simulink model "attitude_interface_sequence"  (R2019b)
settings: Solver=FixedStepAuto  StartTime=0.0  StopTime=inf  FixedStep=FIXED_STEP_SIZE  RelTol=1e-3
model workspace (MAT data in the model file):
  K_ip = 0
  K_pp = 3
values from neighbouring files (symbols this model uses):
  DEG2RAD = pi/180    (= 0.0174532925199)    [attitude_interface_main.m]
  FIXED_STEP_SIZE = 0.01    [attitude_interface_main.m]
  GAZEBO_SYNC_DT = 0.01    [attitude_interface_main.m]
  RAD2DEG = 180/pi    (= 57.2957795131)    [attitude_interface_main.m]
  THRUST_OFFSET = 7.16    [attitude_interface_main.m]
undefined symbols (not defined in the file or in its folder): Header, Pitch, Roll, Thrust, YawRate
libraries: robotlib x5, simulink x3, robotgazebolib x1
settings Model: Creator=ananda  LastModifiedBy=dennis
settings OptimizationCC: EnhancedBackFolding=on  PassReuseOutputArgsAs=Individual arguments  ZeroExternalMemoryAtStartup=off  ZeroInternalMemoryAtStartup=off  MaxStackSize=64  OptimizeBlockOrder=speed  DifferentSizesBufferReuse=on  OptimizationCustomize=off  EfficientTunableParamExpr=on
settings DebuggingCC: ParameterTunabilityLossMsg=error
settings HardwareCC: ProdBitPerPointer=32  ProdBitPerSizeT=32  ProdBitPerPtrDiffT=32  ProdLargestAtomicFloat=None  ProdIntDivRoundTo=Undefined  ProdEndianess=Unspecified  ProdWordSize=32  ProdHWDeviceType=Generic->Unspecified (assume 32-bit Generic)  UseEmbeddedCoderFeatures=off
settings SFSimCC: MATLABDynamicMemAlloc=off
settings RTWCC: SystemTargetFile=ert.tlc  HardwareBoard=Robot Operating System (ROS)  TLCOptions="-aInlineSetEventsForThisBaseRateFcn=TLC_FALSE -aSuppressMultiTaskScheduler=TLC_FALSE  -aRateBasedStepFcn=0"  TemplateMakefile=ert_default_tmf  GenerateReport=on  Toolchain=Catkin  IncludeHyperlinkInReport=on  LaunchReport=on  TargetLang=C++  GenerateTraceInfo=on  GenerateTraceReport=on  GenerateTraceReportSl=on  GenerateTraceReportSf=on  GenerateTraceReportEml=on
settings CodeAppCC: ForceParamTrailComments=on  IgnoreCustomStorageClasses=off  OperatorAnnotations=on  SimulinkDataObjDesc=on  SFDataObjDesc=on  InsertBlockDesc=on
settings ERTTargetCC: SupportNonInlinedSFcns=on

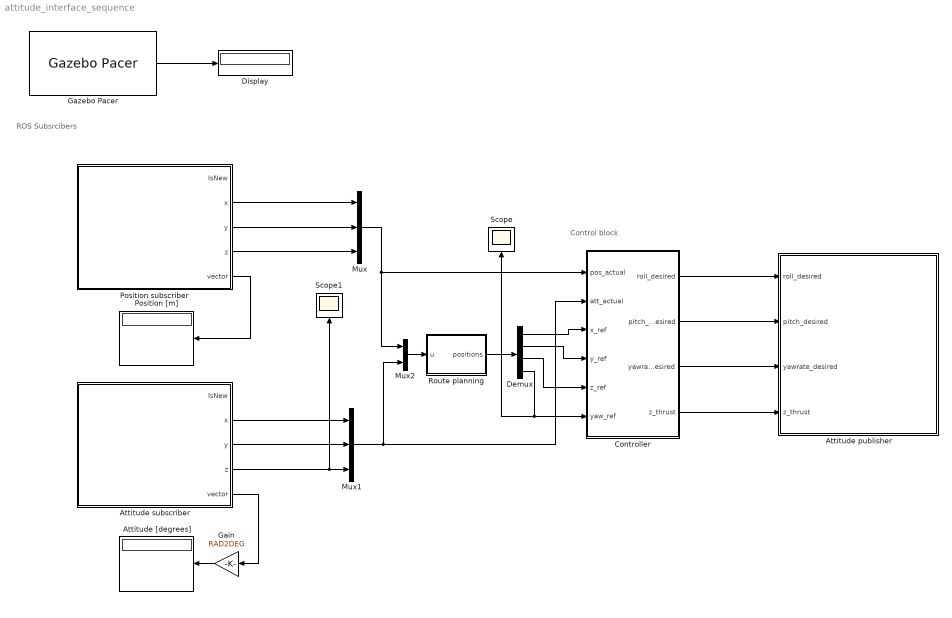
== system attitude_interface_sequence ==
  note: Control block
  note: ROS Subsrcibers
  Attitude [degrees] : Display
  Attitude publisher : Subsystem
  Attitude subscriber : Subsystem
  Controller : Subsystem
  Demux : Demux
  Display : Display
  Gain : Gain  Gain=RAD2DEG
  Gazebo Pacer : robotgazebolib/Gazebo Pacer  ResetBehavior=Reset Gazebo simulation time  SampleTime=GAZEBO_SYNC_DT
      settings: SourceProductName=Robotics System Toolbox  SourceProductBaseCode=RO
  Mux : Mux  Inputs=3
  Mux1 : Mux  Inputs=3
  Mux2 : Mux  Inputs=2
  Position [m] : Display
  Position subscriber : Subsystem
  Route planning : MATLAB Function  TreatAsAtomicUnit=on
      settings: MinAlgLoopOccurrences=on
  Scope : Scope
  Scope1 : Scope
  wires:
  Position subscriber/5(vector) -> Position [m]/1
  Attitude subscriber/5(vector) -> Gain/1
  Gain/1 -> Attitude [degrees]/1
  Gazebo Pacer/1 -> Display/1
  Controller/1(roll_desired) -> Attitude publisher/1(roll_desired)
  Controller/2(pitch_desired) -> Attitude publisher/2(pitch_desired)
  Controller/3(yawrate_desired) -> Attitude publisher/3(yawrate_desired)
  Controller/4(z_thrust) -> Attitude publisher/4(z_thrust)
  Attitude subscriber/2(x) -> Mux1/1
  Attitude subscriber/3(y) -> Mux1/2
  Attitude subscriber/4(z) -> Mux1/3, Scope1/1
  Position subscriber/4(z) -> Mux/3
  Position subscriber/3(y) -> Mux/2
  Position subscriber/2(x) -> Mux/1
  Mux/1 -> Mux2/1, Controller/1(pos_actual)
  Mux1/1 -> Mux2/2, Controller/2(att_actual)
  Mux2/1 -> Route planning/1(u)
  Route planning/1(positions) -> Demux/1
  Demux/1 -> Controller/3(x_ref)
  Demux/2 -> Controller/4(y_ref)
  Demux/3 -> Controller/5(z_ref)
  Demux/4 -> Controller/6(yaw_ref), Scope/1

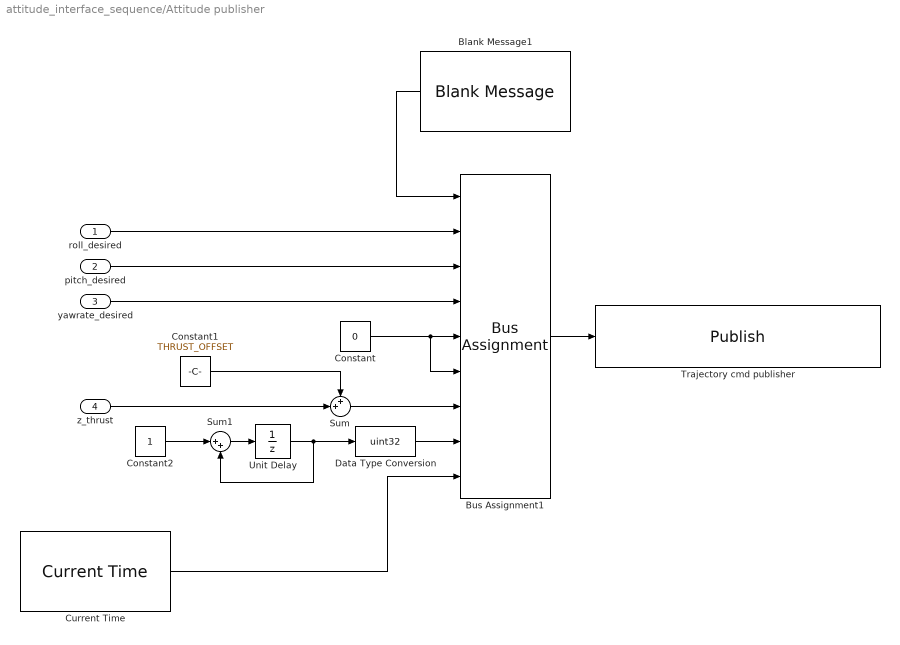
== system attitude_interface_sequence/Attitude publisher ==
  roll_desired : Inport
  pitch_desired : Inport  Port=2
  yawrate_desired : Inport  Port=3
  z_thrust : Inport  Port=4
  Blank Message1 : robotlib/Blank Message  messageClass=Message  entityType=mav_msgs/RollPitchYawrateThrust  messageType=mav_msgs/RollPitchYawrateThrust  SampleTime=FIXED_STEP_SIZE
      settings: SourceProductName=ROS Toolbox
  Bus Assignment1 : BusAssignment  AssignedSignals=Roll,Pitch,YawRate,Thrust.X,Thrust.Y,Thrust.Z,Header.Seq,Header.Stamp
  Constant : Constant  Value=0
  Constant1 : Constant  Value=THRUST_OFFSET
  Constant2 : Constant
  Current Time : robotlib/Current Time  OutputFormat=bus  SampleTime=FIXED_STEP_SIZE  ModelName=attitude_interface_sequence
      settings: SourceProductName=ROS Toolbox  SourceProductBaseCode=RR
  Data Type Conversion : DataTypeConversion  OutDataTypeStr=uint32
  Sum : Sum  Inputs=++|
  Sum1 : Sum  Inputs=|++
  Trajectory cmd publisher : robotlib/Publish  topicSource=Specify your own  topic=/hummingbird/command/roll_pitch_yawrate_thrust  messageType=mav_msgs/RollPitchYawrateThrust  messageQueueLength=1
      settings: SourceProductName=ROS Toolbox
  Unit Delay : UnitDelay  SampleTime=FIXED_STEP_SIZE  HasFrameUpgradeWarning=on
  wires:
  Bus Assignment1/1 -> Trajectory cmd publisher/1
  Blank Message1/1 -> Bus Assignment1/1
  Constant/1 -> Bus Assignment1/6, Bus Assignment1/5
  yawrate_desired/1 -> Bus Assignment1/4
  pitch_desired/1 -> Bus Assignment1/3
  roll_desired/1 -> Bus Assignment1/2
  Sum/1 -> Bus Assignment1/7
  z_thrust/1 -> Sum/2
  Constant1/1 -> Sum/1
  Sum1/1 -> Unit Delay/1
  Unit Delay/1 -> Sum1/2, Data Type Conversion/1
  Constant2/1 -> Sum1/1
  Current Time/1 -> Bus Assignment1/9
  Data Type Conversion/1 -> Bus Assignment1/8

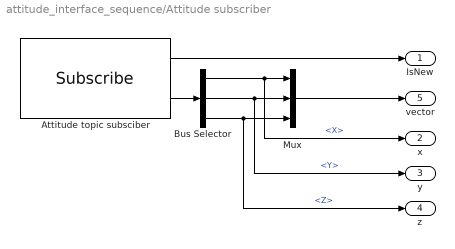
== system attitude_interface_sequence/Attitude subscriber ==
  Attitude topic subsciber : robotlib/Subscribe  topicSource=Specify your own  topic=/hummingbird/orientation_rpy  messageType=geometry_msgs/Vector3  sampleTime=ATTI_SUB_DT  messageQueueLength=1
      settings: SourceProductName=ROS Toolbox
  Bus Selector : BusSelector  OutputSignals=X,Y,Z
  Mux : Mux  Inputs=3
  IsNew : Outport
  x : Outport  Port=2
  y : Outport  Port=3
  z : Outport  Port=4
  vector : Outport  Port=5
  wires:
  Bus Selector/3 -> z/1, Mux/3  "<Z>"
  Bus Selector/2 -> y/1, Mux/2  "<Y>"
  Bus Selector/1 -> x/1, Mux/1  "<X>"
  Attitude topic subsciber/2 -> Bus Selector/1
  Attitude topic subsciber/1 -> IsNew/1
  Mux/1 -> vector/1

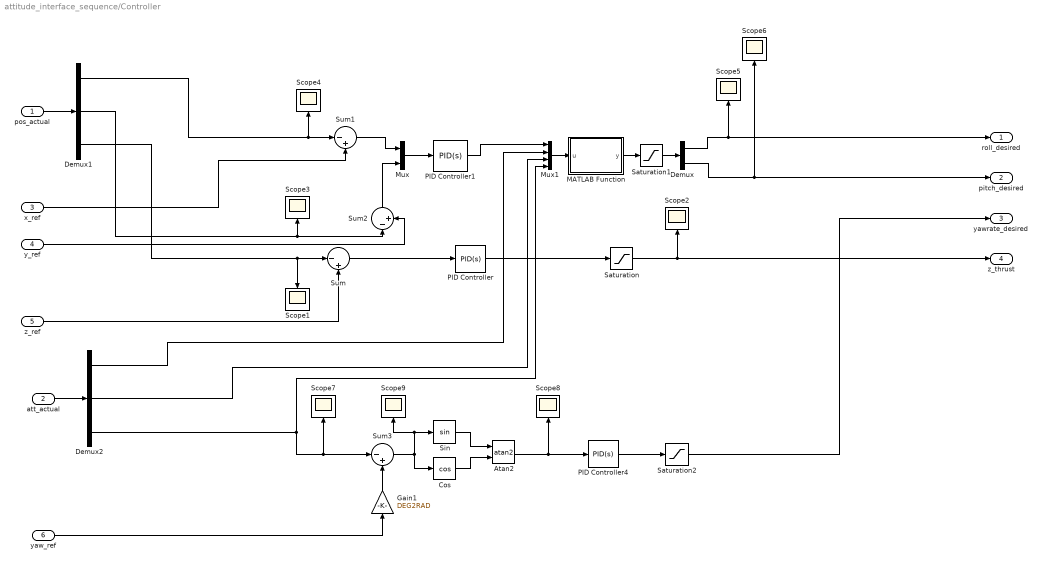
== system attitude_interface_sequence/Controller ==
  pos_actual : Inport
  att_actual : Inport  Port=2
  x_ref : Inport  Port=3
  y_ref : Inport  Port=4
  z_ref : Inport  Port=5
  yaw_ref : Inport  Port=6
  Atan2 : Trigonometry  Operator=atan2
  Cos : Trigonometry  Operator=cos
  Demux : Demux  Outputs=2
  Demux1 : Demux  Outputs=3
  Demux2 : Demux  Outputs=3
  Gain1 : Gain  Gain=DEG2RAD
  MATLAB Function : MATLAB Function  TreatAsAtomicUnit=on
  Mux : Mux  Inputs=2
  Mux1 : Mux
  PID Controller : simulink/Continuous/PID Controller  Controller=PID  Form=Parallel  TimeDomain=Continuous-time  SampleTime=-1  IntegratorMethod=Forward Euler  FilterMethod=Forward Euler  ControllerParametersSource=internal  P=4  I=0.0  D=2.5  UseFilter=on  N=100  TunerSelectOption=Transfer Function Based (PID Tuner App)  InitialConditionSource=internal  InitialConditionForIntegrator=0  InitialConditionForFilter=0  DifferentiatorICPrevScaledInput=0  ExternalReset=none  TrackingMode=off  Kt=1  LimitOutput=off  UpperSaturationLimit=inf  LowerSaturationLimit=-inf  LinearizeAsGain=on  AntiWindupMode=none  Kb=1  POutMin=[]  POutMax=[]  IOutMin=[]  IOutMax=[]  DOutMin=[]  DOutMax=[]  NOutMin=[]  NOutMax=[]  SumOutMin=[]  SumOutMax=[]  SaturationOutMin=[]  SaturationOutMax=[]  PParamMin=[]  PParamMax=[]  IParamMin=[]  IParamMax=[]  DParamMin=[]  DParamMax=[]  NParamMin=[]  NParamMax=[]  KbParamMin=[]  KbParamMax=[]  KtParamMin=[]  KtParamMax=[]  KbOutMin=[]  KbOutMax=[]  KtOutMin=[]  KtOutMax=[]  IntegratorOutMin=[]  IntegratorOutMax=[]  FilterOutMin=[]  FilterOutMax=[]  SumI1OutMin=[]  SumI1OutMax=[]  SumI2OutMin=[]  SumI2OutMax=[]  SumI3OutMin=[]  SumI3OutMax=[]  SumI4OutMin=[]  SumI4OutMax=[]  SumDOutMin=[]  SumDOutMax=[]  DifferentiatorOutMin=[]  DifferentiatorOutMax=[]  FilterDiffOutCoefMin=[]  FilterDiffOutCoefMax=[]  ReciprocalOutMin=[]  ReciprocalOutMax=[]  SumDenOutMin=[]  SumDenOutMax=[]  SumNumOutMin=[]  SumNumOutMax=[]  DivideOutMin=[]  DivideOutMax=[]  IntegratorContinuousStateAttributes=''  IntegratorStateMustResolveToSignalObject=off  IntegratorRTWStateStorageClass=Auto  FilterContinuousStateAttributes=''  FilterStateMustResolveToSignalObject=off  FilterRTWStateStorageClass=Auto  ParallelPVariant=InternalParameters  IdealPVariant=Disabled  IVariant=InternalParameters  DVariant=InternalParameters  IntegratorVariant=Continuous  SatVariant=Disabled  AWVariant=Passthrough  PCopyVariant=Disabled  TRVariant=Disabled  FdbkBlocksVariant=Forward  IdealPFdbkVariant=Disabled  SatFdbkVariant=Disabled  DerivativeFilterVariant=ContFilter  NVariant=InternalParameters  NCopyVariant=Disabled  FilterICVariant=InternalICsFilter  IntegratorICVariant=InternalICs  ExternalResetVariant=Disabled  TRSumVariant=Passthrough  SumFdbkVariant=Disabled  SumVariant=Sum_PID
  PID Controller1 : simulink/Continuous/PID Controller  Controller=PID  Form=Parallel  TimeDomain=Continuous-time  SampleTime=-1  IntegratorMethod=Forward Euler  FilterMethod=Forward Euler  ControllerParametersSource=internal  P=3  I=0.05  D=1.1  UseFilter=on  N=100  TunerSelectOption=Transfer Function Based (PID Tuner App)  InitialConditionSource=internal  InitialConditionForIntegrator=0  InitialConditionForFilter=0  DifferentiatorICPrevScaledInput=0  ExternalReset=none  TrackingMode=off  Kt=1  LimitOutput=off  UpperSaturationLimit=inf  LowerSaturationLimit=-inf  LinearizeAsGain=on  AntiWindupMode=none  Kb=1  POutMin=[]  POutMax=[]  IOutMin=[]  IOutMax=[]  DOutMin=[]  DOutMax=[]  NOutMin=[]  NOutMax=[]  SumOutMin=[]  SumOutMax=[]  SaturationOutMin=[]  SaturationOutMax=[]  PParamMin=[]  PParamMax=[]  IParamMin=[]  IParamMax=[]  DParamMin=[]  DParamMax=[]  NParamMin=[]  NParamMax=[]  KbParamMin=[]  KbParamMax=[]  KtParamMin=[]  KtParamMax=[]  KbOutMin=[]  KbOutMax=[]  KtOutMin=[]  KtOutMax=[]  IntegratorOutMin=[]  IntegratorOutMax=[]  FilterOutMin=[]  FilterOutMax=[]  SumI1OutMin=[]  SumI1OutMax=[]  SumI2OutMin=[]  SumI2OutMax=[]  SumI3OutMin=[]  SumI3OutMax=[]  SumI4OutMin=[]  SumI4OutMax=[]  SumDOutMin=[]  SumDOutMax=[]  DifferentiatorOutMin=[]  DifferentiatorOutMax=[]  FilterDiffOutCoefMin=[]  FilterDiffOutCoefMax=[]  ReciprocalOutMin=[]  ReciprocalOutMax=[]  SumDenOutMin=[]  SumDenOutMax=[]  SumNumOutMin=[]  SumNumOutMax=[]  DivideOutMin=[]  DivideOutMax=[]  IntegratorContinuousStateAttributes=''  IntegratorStateMustResolveToSignalObject=off  IntegratorRTWStateStorageClass=Auto  FilterContinuousStateAttributes=''  FilterStateMustResolveToSignalObject=off  FilterRTWStateStorageClass=Auto  ParallelPVariant=InternalParameters  IdealPVariant=Disabled  IVariant=InternalParameters  DVariant=InternalParameters  IntegratorVariant=Continuous  SatVariant=Disabled  AWVariant=Passthrough  PCopyVariant=Disabled  TRVariant=Disabled  FdbkBlocksVariant=Forward  IdealPFdbkVariant=Disabled  SatFdbkVariant=Disabled  DerivativeFilterVariant=ContFilter  NVariant=InternalParameters  NCopyVariant=Disabled  FilterICVariant=InternalICsFilter  IntegratorICVariant=InternalICs  ExternalResetVariant=Disabled  TRSumVariant=Passthrough  SumFdbkVariant=Disabled  SumVariant=Sum_PID
  PID Controller4 : simulink/Continuous/PID Controller  Controller=PID  Form=Parallel  TimeDomain=Continuous-time  SampleTime=-1  IntegratorMethod=Forward Euler  FilterMethod=Forward Euler  ControllerParametersSource=internal  P=4  I=0.3  D=1.5  UseFilter=on  N=100  TunerSelectOption=Transfer Function Based (PID Tuner App)  InitialConditionSource=internal  InitialConditionForIntegrator=0  InitialConditionForFilter=0  DifferentiatorICPrevScaledInput=0  ExternalReset=none  TrackingMode=off  Kt=1  LimitOutput=off  UpperSaturationLimit=inf  LowerSaturationLimit=-inf  LinearizeAsGain=on  AntiWindupMode=none  Kb=1  POutMin=[]  POutMax=[]  IOutMin=[]  IOutMax=[]  DOutMin=[]  DOutMax=[]  NOutMin=[]  NOutMax=[]  SumOutMin=[]  SumOutMax=[]  SaturationOutMin=[]  SaturationOutMax=[]  PParamMin=[]  PParamMax=[]  IParamMin=[]  IParamMax=[]  DParamMin=[]  DParamMax=[]  NParamMin=[]  NParamMax=[]  KbParamMin=[]  KbParamMax=[]  KtParamMin=[]  KtParamMax=[]  KbOutMin=[]  KbOutMax=[]  KtOutMin=[]  KtOutMax=[]  IntegratorOutMin=[]  IntegratorOutMax=[]  FilterOutMin=[]  FilterOutMax=[]  SumI1OutMin=[]  SumI1OutMax=[]  SumI2OutMin=[]  SumI2OutMax=[]  SumI3OutMin=[]  SumI3OutMax=[]  SumI4OutMin=[]  SumI4OutMax=[]  SumDOutMin=[]  SumDOutMax=[]  DifferentiatorOutMin=[]  DifferentiatorOutMax=[]  FilterDiffOutCoefMin=[]  FilterDiffOutCoefMax=[]  ReciprocalOutMin=[]  ReciprocalOutMax=[]  SumDenOutMin=[]  SumDenOutMax=[]  SumNumOutMin=[]  SumNumOutMax=[]  DivideOutMin=[]  DivideOutMax=[]  IntegratorContinuousStateAttributes=''  IntegratorStateMustResolveToSignalObject=off  IntegratorRTWStateStorageClass=Auto  FilterContinuousStateAttributes=''  FilterStateMustResolveToSignalObject=off  FilterRTWStateStorageClass=Auto  ParallelPVariant=InternalParameters  IdealPVariant=Disabled  IVariant=InternalParameters  DVariant=InternalParameters  IntegratorVariant=Continuous  SatVariant=Disabled  AWVariant=Passthrough  PCopyVariant=Disabled  TRVariant=Disabled  FdbkBlocksVariant=Forward  IdealPFdbkVariant=Disabled  SatFdbkVariant=Disabled  DerivativeFilterVariant=ContFilter  NVariant=InternalParameters  NCopyVariant=Disabled  FilterICVariant=InternalICsFilter  IntegratorICVariant=InternalICs  ExternalResetVariant=Disabled  TRSumVariant=Passthrough  SumFdbkVariant=Disabled  SumVariant=Sum_PID
  Saturation : Saturate  UpperLimit=15  LowerLimit=-15
  Saturation1 : Saturate  LinearizeAsGain=off
  Saturation2 : Saturate  UpperLimit=8  LowerLimit=-8
  Scope{1..9} (9 alike) : Scope
  Sin : Trigonometry
  Sum{,1..3} (4 alike) : Sum  Inputs=|-+
  roll_desired : Outport
  pitch_desired : Outport  Port=2
  yawrate_desired : Outport  Port=3
  z_thrust : Outport  Port=4
  wires:
  PID Controller4/1 -> Saturation2/1
  Gain1/1 -> Sum3/2
  Sum1/1 -> Mux/1
  Cos/1 -> Atan2/2
  Demux2/3 -> Sum3/1, Scope7/1, Mux1/4
  x_ref/1 -> Sum1/2
  Saturation2/1 -> yawrate_desired/1
  Demux1/1 -> Sum1/1, Scope4/1
  Demux1/3 -> Sum/1, Scope1/1
  Demux2/2 -> Mux1/3
  Sum2/1 -> Mux/2
  Atan2/1 -> Scope8/1, PID Controller4/1
  Mux/1 -> PID Controller1/1
  yaw_ref/1 -> Gain1/1
  Demux1/2 -> Sum2/1, Scope3/1
  Demux/2 -> pitch_desired/1, Scope6/1
  PID Controller/1 -> Saturation/1
  Demux2/1 -> Mux1/2
  PID Controller1/1 -> Mux1/1
  Demux/1 -> roll_desired/1, Scope5/1
  Mux1/1 -> MATLAB Function/1(u)
  Saturation/1 -> z_thrust/1, Scope2/1
  Sum3/1 -> Cos/1, Sin/1, Scope9/1
  MATLAB Function/1(y) -> Saturation1/1
  y_ref/1 -> Sum2/2
  Saturation1/1 -> Demux/1
  Sin/1 -> Atan2/1
  Sum/1 -> PID Controller/1
  z_ref/1 -> Sum/2
  pos_actual/1 -> Demux1/1
  att_actual/1 -> Demux2/1

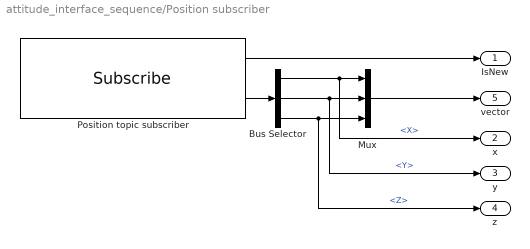
== system attitude_interface_sequence/Position subscriber ==
  Bus Selector : BusSelector  OutputSignals=Point.X,Point.Y,Point.Z
  Mux : Mux  Inputs=3
  Position topic subscriber : robotlib/Subscribe  topicSource=Specify your own  topic=/hummingbird/odometry_sensor1/position  messageType=geometry_msgs/PointStamped  sampleTime=POS_SUB_DT  messageQueueLength=1
      settings: SourceProductName=ROS Toolbox
  IsNew : Outport
  x : Outport  Port=2
  y : Outport  Port=3
  z : Outport  Port=4
  vector : Outport  Port=5
  wires:
  Bus Selector/3 -> z/1, Mux/3  "<Z>"
  Bus Selector/2 -> y/1, Mux/2  "<Y>"
  Mux/1 -> vector/1
  Bus Selector/1 -> x/1, Mux/1  "<X>"
  Position topic subscriber/2 -> Bus Selector/1
  Position topic subscriber/1 -> IsNew/1

== matlab function attitude_interface_sequence/Route planning ==
  data: u input; positions output
function positions = fcn(u)

persistent count;

meas_x = u(1);
meas_y = u(2);
meas_alt = u(3);
meas_psi = u(6);

reference = [meas_x, meas_y, meas_alt]';

if (isempty(count))
    count = 0;
end

route = [0, 0, 1; 2, 0, 1; 2, 2, 1; 0, 2, 1; 0, 0, 0]';
yaw = [0; 90; 180; -90; 0]';

idx = mod(count,length(route)) + 1;

pos = [route(1, idx), route(2, idx), route(3, idx)]';
posediff = norm(pos-reference);
yawdiff = deg2rad(yaw(idx)) - meas_psi;
poseyawdiff = atan2(sin(yawdiff), cos(yawdiff));

if posediff < 0.05 && abs(poseyawdiff) < 1 * pi/180
    count = count + 1;
    idx = mod(count,length(route)) + 1;
end

positions = [route(1, idx), route(2, idx), route(3, idx), yaw(idx)]';

end

== matlab function attitude_interface_sequence/Controller/MATLAB Function ==
  data: u input; y output
function y = fcn(u)

ex = u(1);
ey = u(2);
phi = u(3);
theta = u(4);
psi = u(5);

y = [ex*(cos(phi)*sin(psi) - cos(psi)*sin(phi)*sin(theta)) - ey*(cos(phi)*cos(psi) + sin(phi)*sin(psi)*sin(theta));
     ex*cos(psi)*cos(theta) + ey*cos(theta)*sin(psi)];

end
